simulink model "sistema_di_controllo_digitale_rev3_1"  (Simulink 7.7)
settings: Solver=ode3  StartTime=0.0  StopTime=2*stop_t  FixedStep=Ts  MaxStep=Ts/10  MinStep=Ts/100  RelTol=1e-3
values from neighbouring files (symbols this model uses):
  a_da = 0    [CA_GIUSE.m]    (also in Script.m)
  a_dp = 0e-2    (= 0)    [CA_GIUSE.m]    (also in Script.m)
  a_ds = 0e-2    (= 0)    [CA_GIUSE.m]    (also in Script.m)
  AA_order = 2    [CA_GIUSE.m]    (also in Script.m)
  aph = 0.00    (= 0)    [CA_GIUSE.m]    (also in Script.m = 0.05)
  Da_c = 0e-3    (= 0)    [CA_GIUSE.m]    (also in Script.m)
  Da_r = 0    [CA_GIUSE.m]    (also in Script.m)
  Dp_c = 0e-4    (= 0)    [CA_GIUSE.m]    (also in Script.m)
  Dp_r = 0    [CA_GIUSE.m]    (also in Script.m)
  Ds_c = 0    [CA_GIUSE.m]    (also in Script.m)
  Ds_r = 0    [CA_GIUSE.m]    (also in Script.m)
  Ga = 0e3    (= 0)    [CA_GIUSE.m]    (also in Script.m)
  Gda = 1    [CA_GIUSE.m]    (also in Script.m)
  Gf = 1/(Kd*Gs)    [CA_GIUSE.m]    (also in Script.m)
  Gr = 0    [CA_GIUSE.m]    (also in Script.m = 1)
  Gs =     [CA_GIUSE.m]    (also in Script.m = 0)
  Kd =     [CA_GIUSE.m]    (also in Script.m = 0)
  over = 0.0    (= 0)    [CA_GIUSE.m]    (also in Script.m)
  Pulse_da = 0    [CA_GIUSE.m]    (also in Script.m)
  Pulse_dp = 0e-0    (= 0)    [CA_GIUSE.m]    (also in Script.m)
  Pulse_ds = 0    [CA_GIUSE.m]    (also in Script.m)
  R_0 = 1    [CA_GIUSE.m]    (also in Script.m)
  sig_gen_amp = 1    [CA_GIUSE.m]    (also in Script.m = 0.5)
  sig_gen_freq = 0.5    [CA_GIUSE.m]    (also in Script.m = 0.25)
  Ts = 0.1/(Wceff)    [CA_GIUSE.m]    (also in Script.m = 0.1/(Wceff); [Gcz,Lz]=TDmode(Ts,Glp,Gc,Ga,Gp,Gs,Gf))
undefined symbols (not defined in the file or in its folder): den_Gcz, den_Gp, num_Gcz, num_Gp
libraries: simulink x20, dsparch4 x1
settings Model: Creator=Sandro  LastModifiedBy=giuse

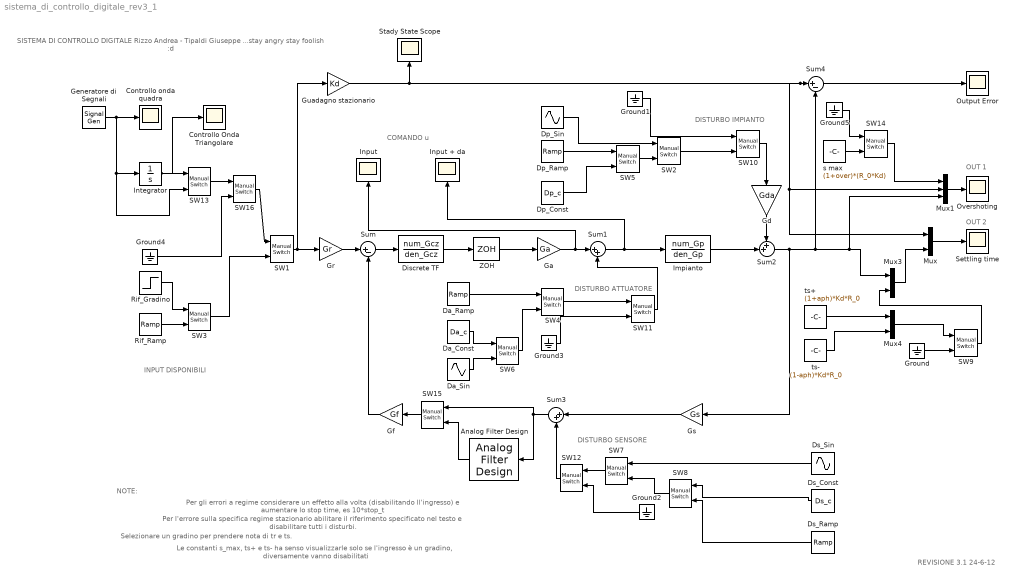
== system sistema_di_controllo_digitale_rev3_1 ==
  note: SISTEMA DI CONTROLLO DIGITALE
      | Rizzo Andrea - Tipaldi Giuseppe
      |
      | ...stay angry stay foolish
      | :d
  note: DISTURBO ATTUATORE
  note: DISTURBO IMPIANTO
  note: INPUT DISPONIBILI
  note: COMANDO u
  note: DISTURBO SENSORE
  note: OUT 1
  note: OUT 2
  note: NOTE:
  note: Per gli errori a regime considerare un effetto alla volta (disabilitando ll'ingresso) e aumentare lo stop time, es 10*stop_t
  note: Selezionare un gradino per prendere nota di tr e ts.
  note: Per l'errore sulla specifica regime stazionario abilitare il riferimento specificato nel testo e disabilitare tutti i disturbi.
  note: Le constanti s_max, ts+ e ts- ha senso visualizzarle solo se l'ingresso è un gradino, diversamente vanno disabilitati
  note: REVISIONE 3.1 24-6-12
  " s max" : Constant  Value=(1+over)*(R_0*Kd)
  Analog Filter Design : dsparch4/Analog Filter Design  method=Bessel  filttype=Lowpass  N=AA_order  Wlo=Pulse_AAF  Whi=80  Rp=2  Rs=40
  Controllo Onda Triangolare : Scope
      settings: SaveName=ScopeData3
  Controllo onda quadra : Scope
      settings: TimeRange=0.002216033935546875  YMin=2.1909418072197  YMax=2.191153294711311  SaveName=ScopeData6
  Da_Const : Constant  Value=Da_c
  Da_Ramp : simulink/Sources/Ramp  SystemSampleTime=-1  slope=Da_r  start=0  X0=0
  Da_Sin : Sin  Amplitude=a_da  Frequency=Pulse_da  SampleTime=0
  Discrete TF : DiscreteTransferFcn  Numerator=num_Gcz  Denominator=den_Gcz  SampleTime=Ts
  Dp_Const : Constant  Value=Dp_c
  Dp_Ramp : simulink/Sources/Ramp  SystemSampleTime=-1  slope=Dp_r  start=0  X0=0
  Dp_Sin : Sin  Amplitude=a_dp  Frequency=Pulse_dp  SampleTime=0
  Ds_Const : Constant  Value=Ds_c
  Ds_Ramp : simulink/Sources/Ramp  SystemSampleTime=-1  slope=Ds_r  start=0  X0=0
  Ds_Sin : Sin  Amplitude=a_ds  Frequency=Pulse_ds  SampleTime=0
  Ga : Gain  Gain=Ga
  Gd : Gain  Gain=Gda
  Generatore di Segnali : SignalGenerator  WaveForm=square  Amplitude=sig_gen_amp  Frequency=sig_gen_freq  Units=rad/sec
  Gf : Gain  Gain=Gf
  Gr : Gain  Gain=Gr
  Ground{,1..5} (6 alike) : Ground
  Gs : Gain  Gain=Gs
  Guadagno stazionario : Gain  Gain=Kd
  Impianto : TransferFcn  Numerator=num_Gp  Denominator=den_Gp
  Input : Scope
      settings: TimeRange=7.62942779291553  YMin=0.9536585365853658  YMax=1.036585365853659  SaveName=ScopeData4
  Input + da : Scope
      settings: TimeRange=7.62942779291553  YMin=0.9536585365853658  YMax=1.036585365853659
  Integrator : Integrator  InitialCondition=0.5
  Mux : Mux  Inputs=2
  Mux1 : Mux  Inputs=3
  Mux3 : Mux  Inputs=2
  Mux4 : Mux  Inputs=2
  Output Error : Scope
      settings: TimeRange=2  YMin=-0.003785942087987625  YMax=-0.003563613211040456  SaveName=ScopeData2
  Overshoting : Scope
      settings: TimeRange=0.003554270833333334  YMin=1.975  YMax=2.4  SaveName=ScopeData5
  Rif_Gradino : Step  Time=0  After=R_0  SampleTime=0
  Rif_Ramp : simulink/Sources/Ramp  SystemSampleTime=-1  slope=R_0  start=0  X0=0
  SW{1..2,4..5,11..14,16} (9 alike) : simulink/Signal Routing/Manual Switch  SystemSampleTime=-1  sw=0  action=0  varsize=off
  SW{3,6..10,15} (7 alike) : simulink/Signal Routing/Manual Switch  SystemSampleTime=-1  sw=1  action=0  varsize=off
  Settling time : Scope
      settings: TimeRange=1.6  YMin=-3.580716253443526e+244  YMax=-3.80716253443527e+243
  Stady State Scope : Scope
      settings: TimeRange=7.62942779291553  YMin=0.9536585365853658  YMax=1.036585365853659  SaveName=ScopeData7
  Sum : Sum  Inputs=|+-
  Sum1 : Sum  Inputs=|++
  Sum2 : Sum  Inputs=++|
  Sum3 : Sum  Inputs=|++
  Sum4 : Sum  Inputs=|+-
  ZOH : ZeroOrderHold  SampleTime=Ts
  ts+ : Constant  Value=(1+aph)*Kd*R_0
  ts- : Constant  Value=(1-aph)*Kd*R_0
  wires:
  Sum1/1 -> Impianto/1, Input + da/1
  Sum2/1 -> Gs/1, Mux3/1, Mux1/3, Sum4/2
  Guadagno stazionario/1 -> Sum4/1, Mux/1, Mux1/2, Stady State Scope/1
  Mux/1 -> Settling time/1
  Impianto/1 -> Sum2/2
  Gd/1 -> Sum2/1
  Gs/1 -> Sum3/1
  Gr/1 -> Sum/1
  SW3/1 -> SW1/2
  SW5/1 -> SW2/2
  SW6/1 -> SW4/2
  Dp_Const/1 -> SW5/2
  Dp_Sin/1 -> SW2/1
  Dp_Ramp/1 -> SW5/1
  Da_Sin/1 -> SW6/2
  Da_Const/1 -> SW6/1
  Da_Ramp/1 -> SW4/1
  Rif_Ramp/1 -> SW3/2
  Rif_Gradino/1 -> SW3/1
  SW8/1 -> SW7/2
  Ds_Sin/1 -> SW7/1
  Ds_Const/1 -> SW8/1
  Ds_Ramp/1 -> SW8/2
  Sum4/1 -> Output Error/1
  ts-/1 -> Mux4/2
  ts+/1 -> Mux4/1
  Mux4/1 -> SW9/1
  SW9/1 -> Mux3/2
  Ground/1 -> SW9/2
  Mux1/1 -> Overshoting/1
  SW2/1 -> SW10/2
  SW10/1 -> Gd/1
  Ground1/1 -> SW10/1
  SW7/1 -> SW12/1
  SW12/1 -> Sum3/2
  Ground2/1 -> SW12/2
  SW4/1 -> SW11/1
  Ground3/1 -> SW11/2
  SW11/1 -> Sum1/2
  Generatore di Segnali/1 -> Controllo onda quadra/1, SW13/2, Integrator/1
  Mux3/1 -> Mux/2
  SW1/1 -> Gr/1, Guadagno stazionario/1
  Sum3/1 -> SW15/1, Analog Filter Design/1
  Gf/1 -> Sum/2
  " s max"/1 -> SW14/2
  SW14/1 -> Mux1/1
  Ground5/1 -> SW14/1
  SW15/1 -> Gf/1
  Analog Filter Design/1 -> SW15/2
  Discrete TF/1 -> ZOH/1
  ZOH/1 -> Ga/1
  Sum/1 -> Discrete TF/1
  Ga/1 -> Sum1/1, Input/1
  SW13/1 -> SW16/1
  Ground4/1 -> SW16/2
  SW16/1 -> SW1/1
  Integrator/1 -> Controllo Onda Triangolare/1, SW13/1
